simulink model "test_kin_odwrotnej"  (Simulink 7.7)
settings: Solver=FixedStepDiscrete  StartTime=0.0  StopTime=0  FixedStep=1  RelTol=1e-3
values from neighbouring files (symbols this model uses):
  Rmax = 947    [kin_odwr.mat]    (also in test_kin_odwr_ost.m = 945)
  Rmin = 461    [kin_odwr.mat]    (also in test_kin_odwr_ost.m = 463)
  wsp_x = 1010    [kin_odwr.mat]    (also in test_kin_odwr_ost.m = (j-100)*10)
  wsp_y = 2610    [kin_odwr.mat]    (also in test_kin_odwr_ost.m = (i-100)*10)
  wsp_z = 930    [kin_odwr.mat]    (also in test_kin_odwr.m; test_kin_odwr_ost.m)
  y_akt = 0    [kin_odwr.mat]    (also in test_kin_odwr_ost.m)
undefined symbols (not defined in the file or in its folder): sgn
libraries: simulink x27, simulink_extras x4
settings Model: Creator=Maciek  LastModifiedBy=Maciek

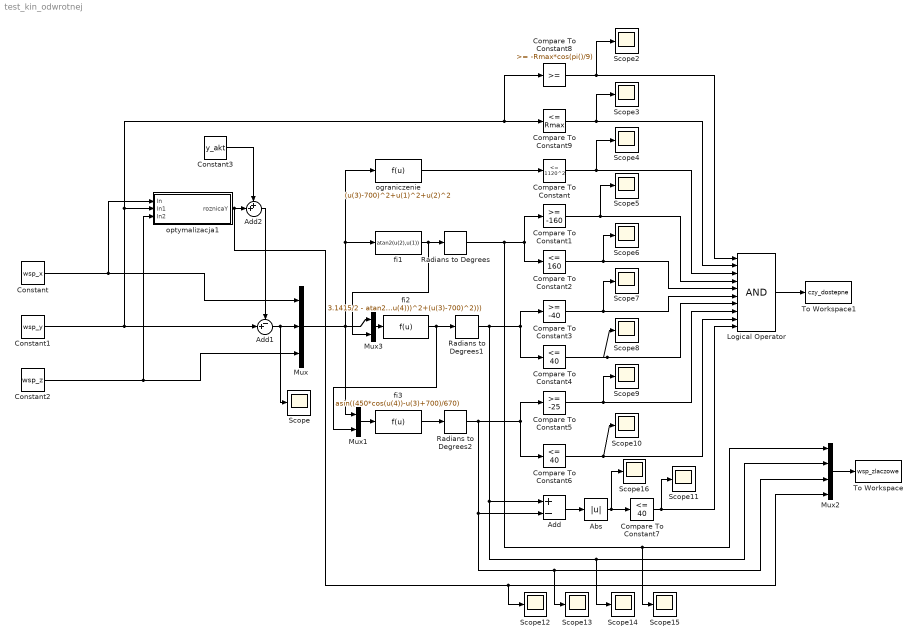
== system test_kin_odwrotnej ==
  Abs : Abs
  Add : Sum  Inputs=+-
  Add1 : Sum  Inputs=-+|
  Add2 : Sum  Inputs=++|
  Compare To Constant : simulink/Logic and Bit Operations/Compare To Constant  SystemSampleTime=-1  relop=<=  const=1120^2  LogicOutDataTypeMode=boolean  ZeroCross=off
  Compare To Constant1 : simulink/Logic and Bit Operations/Compare To Constant  SystemSampleTime=-1  relop=>=  const=-160  LogicOutDataTypeMode=boolean  ZeroCross=off
  Compare To Constant2 : simulink/Logic and Bit Operations/Compare To Constant  SystemSampleTime=-1  relop=<=  const=160  LogicOutDataTypeMode=boolean  ZeroCross=off
  Compare To Constant3 : simulink/Logic and Bit Operations/Compare To Constant  SystemSampleTime=-1  relop=>=  const=-40  LogicOutDataTypeMode=boolean  ZeroCross=off
  Compare To Constant4 : simulink/Logic and Bit Operations/Compare To Constant  SystemSampleTime=-1  relop=<=  const=40  LogicOutDataTypeMode=boolean  ZeroCross=off
  Compare To Constant5 : simulink/Logic and Bit Operations/Compare To Constant  SystemSampleTime=-1  relop=>=  const=-25  LogicOutDataTypeMode=boolean  ZeroCross=off
  Compare To Constant6 : simulink/Logic and Bit Operations/Compare To Constant  SystemSampleTime=-1  relop=<=  const=40  LogicOutDataTypeMode=boolean  ZeroCross=off
  Compare To Constant7 : simulink/Logic and Bit Operations/Compare To Constant  SystemSampleTime=-1  relop=<=  const=40  LogicOutDataTypeMode=boolean  ZeroCross=off
  Compare To Constant8 : simulink/Logic and Bit Operations/Compare To Constant  SystemSampleTime=-1  relop=>=  const=-Rmax*cos(pi()/9)  LogicOutDataTypeMode=boolean  ZeroCross=off
  Compare To Constant9 : simulink/Logic and Bit Operations/Compare To Constant  SystemSampleTime=-1  relop=<=  const=Rmax  LogicOutDataTypeMode=boolean  ZeroCross=off
  Constant : Constant  Value=wsp_x
  Constant1 : Constant  Value=wsp_y
  Constant2 : Constant  Value=wsp_z
  Constant3 : Constant  Value=y_akt  OutDataTypeStr=double
  Logical Operator : Logic  Inputs=10  AllPortsSameDT=off  OutDataTypeStr=boolean
  Mux : Mux  Inputs=3
  Mux1 : Mux  Inputs=2
  Mux2 : Mux
  Mux3 : Mux  Inputs=2
  Radians to Degrees : simulink_extras/Transformations/Radians to Degrees  SystemSampleTime=-1
  Radians to Degrees1 : simulink_extras/Transformations/Radians to Degrees  SystemSampleTime=-1
  Radians to Degrees2 : simulink_extras/Transformations/Radians to Degrees  SystemSampleTime=-1
  Scope{,2..16} (16 alike) : Scope
      Scope settings: SaveName=ScopeData18
      Scope10 settings: SaveName=ScopeData35
      Scope11 settings: SaveName=ScopeData36
      Scope12 settings: SaveName=ScopeData37
      Scope13 settings: SaveName=ScopeData38
      Scope14 settings: SaveName=ScopeData39
      Scope15 settings: SaveName=ScopeData40
      Scope16 settings: SaveName=ScopeData47
      Scope2 settings: SaveName=ScopeData27
      Scope3 settings: SaveName=ScopeData28
      Scope4 settings: SaveName=ScopeData29
      Scope5 settings: SaveName=ScopeData30
      Scope6 settings: SaveName=ScopeData31
      Scope7 settings: SaveName=ScopeData32
      Scope8 settings: SaveName=ScopeData33
      Scope9 settings: SaveName=ScopeData34
  To Workspace : ToWorkspace  VariableName=wsp_zlaczowe  SampleTime=-1  SaveFormat=Array
  To Workspace1 : ToWorkspace  VariableName=czy_dostepne  SampleTime=-1  SaveFormat=Array
  fi1 : Fcn  Expr=atan2(u(2),u(1))
  fi2 : Fcn  Expr=3.1415/2 - atan2((u(3)-700),sqrt((u(1)-cos(u(4))*250)^2+(u(2)-250*sin(u(4)))^2)) - acos((450^2+(u(1)-250*cos(u(4)))^2+(u(2)-250*sin(u(4)))^2+(u(3)-700)^2-670^2)/(2*450*sqrt((u(1)-250*cos(u(4)))^2+(u(2)-250*sin(u(4)))^2+(u(3)-700)^2)))
  fi3 : Fcn  Expr=asin((450*cos(u(4))-u(3)+700)/670)
  ograniczenie : Fcn  Expr=(u(3)-700)^2+u(1)^2+u(2)^2
  optymalizacja1 : Subsystem
  wires:
  fi1/1 -> Radians to Degrees/1, Mux3/2
  ograniczenie/1 -> Compare To Constant/1
  Radians to Degrees/1 -> Compare To Constant1/1, Compare To Constant2/1, Mux2/1, Scope15/1
  Add/1 -> Abs/1
  Abs/1 -> Compare To Constant7/1, Scope16/1
  Radians to Degrees1/1 -> Compare To Constant3/1, Compare To Constant4/1, Add/1, Mux2/2, Scope14/1
  fi3/1 -> Radians to Degrees2/1
  fi2/1 -> Radians to Degrees1/1, Mux1/2
  Radians to Degrees2/1 -> Compare To Constant5/1, Compare To Constant6/1, Add/2, Scope13/1, Mux2/3
  Compare To Constant7/1 -> Logical Operator/10, Scope11/1
  Compare To Constant/1 -> Logical Operator/3, Scope4/1
  Compare To Constant1/1 -> Logical Operator/4, Scope5/1
  Compare To Constant2/1 -> Logical Operator/5, Scope6/1
  Compare To Constant3/1 -> Logical Operator/6, Scope7/1
  Compare To Constant4/1 -> Logical Operator/7, Scope8/1
  Compare To Constant5/1 -> Logical Operator/8, Scope9/1
  Compare To Constant6/1 -> Logical Operator/9, Scope10/1
  Mux1/1 -> fi3/1
  Mux/1 -> ograniczenie/1, fi1/1, Mux1/1, Mux3/1
  Constant2/1 -> Mux/3, optymalizacja1/3(In2)
  Constant1/1 -> optymalizacja1/2(In1), Compare To Constant9/1, Compare To Constant8/1, Add1/2
  Compare To Constant9/1 -> Logical Operator/2, Scope3/1
  Compare To Constant8/1 -> Logical Operator/1, Scope2/1
  Mux2/1 -> To Workspace/1
  Constant/1 -> optymalizacja1/1(In), Mux/1
  Add1/1 -> Mux/2, Scope/1
  Logical Operator/1 -> To Workspace1/1
  optymalizacja1/1(roznicaY) -> Add2/2, Mux2/4, Scope12/1
  Add2/1 -> Add1/1
  Constant3/1 -> Add2/1
  Mux3/1 -> fi2/1

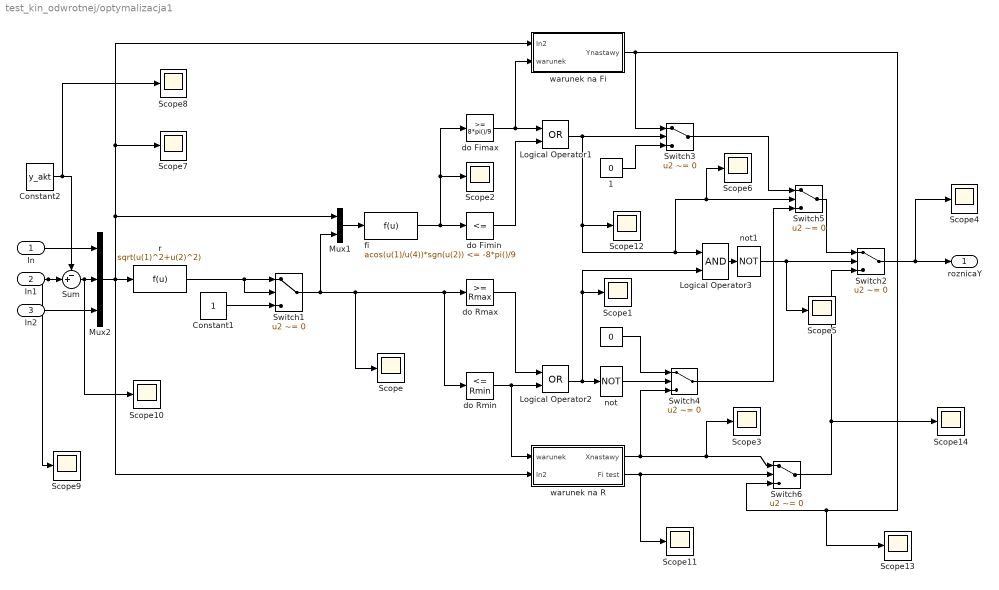
== system test_kin_odwrotnej/optymalizacja1 ==
  In : Inport
  In1 : Inport  Port=2
  In2 : Inport  Port=3
  " " : Constant  Value=0  OutDataTypeStr=double
  " 1" : Constant  Value=0  OutDataTypeStr=double
  Constant1 : Constant  OutDataTypeStr=double
  Constant2 : Constant  Value=y_akt  OutDataTypeStr=double
  Logical Operator1 : Logic  Operator=OR  AllPortsSameDT=off  OutDataTypeStr=boolean
  Logical Operator2 : Logic  Operator=OR  AllPortsSameDT=off  OutDataTypeStr=boolean
  Logical Operator3 : Logic  AllPortsSameDT=off  OutDataTypeStr=boolean
  Mux1 : Mux  Inputs=2
  Mux2 : Mux  Inputs=3
  Scope{,1..14} (15 alike) : Scope
      Scope10 settings: SaveName=ScopeData46
      Scope11 settings: SaveName=ScopeData50
      Scope12 settings: SaveName=ScopeData51
      Scope13 settings: SaveName=ScopeData53
      Scope14 settings: SaveName=ScopeData54
      Scope2 settings: SaveName=ScopeData2
      Scope3 settings: SaveName=ScopeData3
      Scope4 settings: SaveName=ScopeData16
      Scope5 settings: SaveName=ScopeData17
      Scope6 settings: SaveName=ScopeData41
      Scope7 settings: SaveName=ScopeData43
      Scope8 settings: SaveName=ScopeData44
      Scope9 settings: SaveName=ScopeData45
  Sum : Sum  Inputs=-+|
  Switch1 : Switch  Criteria=u2 ~= 0  OutDataTypeStr=double
  Switch{2..6} (5 alike) : Switch  Criteria=u2 ~= 0
  do Fimax : simulink/Logic and Bit Operations/Compare To Constant  SystemSampleTime=-1  relop=>=  const=8*pi()/9  LogicOutDataTypeMode=uint8  ZeroCross=off
  do Fimin : simulink/Logic and Bit Operations/Compare To Constant  SystemSampleTime=-1  relop=<=  const=-8*pi()/9  LogicOutDataTypeMode=uint8  ZeroCross=off
  do Rmax : simulink/Logic and Bit Operations/Compare To Constant  SystemSampleTime=-1  relop=>=  const=Rmax  LogicOutDataTypeMode=uint8  ZeroCross=off
  do Rmin : simulink/Logic and Bit Operations/Compare To Constant  SystemSampleTime=-1  relop=<=  const=Rmin  LogicOutDataTypeMode=uint8  ZeroCross=off
  fi : Fcn  Expr=acos(u(1)/u(4))*sgn(u(2))
  not : Logic  Operator=NOT  AllPortsSameDT=off  OutDataTypeStr=boolean
  not1 : Logic  Operator=NOT  AllPortsSameDT=off  OutDataTypeStr=boolean
  r : Fcn  Expr=sqrt(u(1)^2+u(2)^2)
  warunek na Fi : Subsystem  TreatAsAtomicUnit=on
  warunek na R : Subsystem  TreatAsAtomicUnit=on
  roznicaY : Outport
  wires:
  Switch6/1 -> Switch2/3, Scope14/1
  warunek na R/2(Fi test) -> Switch6/2, Scope11/1
  not1/1 -> Switch2/2, Scope5/1
  Switch3/1 -> Switch5/1
  Switch4/1 -> Switch5/3
  Switch5/1 -> Switch2/1
  Logical Operator3/1 -> not1/1
  " 1"/1 -> Switch3/3
  " "/1 -> Switch4/1
  not/1 -> Switch4/2
  warunek na R/1(Xnastawy) -> Switch4/3, Switch6/1, Scope3/1
  warunek na Fi/1(Ynastawy) -> Switch3/1, Switch6/3, Scope13/1
  Logical Operator1/1 -> Switch3/2, Logical Operator3/1, Switch5/2, Scope6/1, Scope12/1
  Logical Operator2/1 -> not/1, Logical Operator3/2, Scope1/1
  do Rmin/1 -> Logical Operator2/2, warunek na R/1(warunek)
  do Rmax/1 -> Logical Operator2/1
  do Fimin/1 -> Logical Operator1/2
  do Fimax/1 -> warunek na Fi/2(warunek), Logical Operator1/1
  fi/1 -> do Fimin/1, do Fimax/1, Scope2/1
  Constant1/1 -> Switch1/3
  Mux1/1 -> fi/1
  Switch1/1 -> Mux1/2, do Rmax/1, do Rmin/1, Scope/1
  r/1 -> Switch1/2, Switch1/1
  Mux2/1 -> r/1, Mux1/1, warunek na Fi/1(In2), Scope7/1, warunek na R/2(In2)
  In/1 -> Mux2/1
  In2/1 -> Mux2/3
  Switch2/1 -> roznicaY/1, Scope4/1
  Sum/1 -> Mux2/2, Scope10/1
  In1/1 -> Sum/2, Scope9/1
  Constant2/1 -> Sum/1, Scope8/1

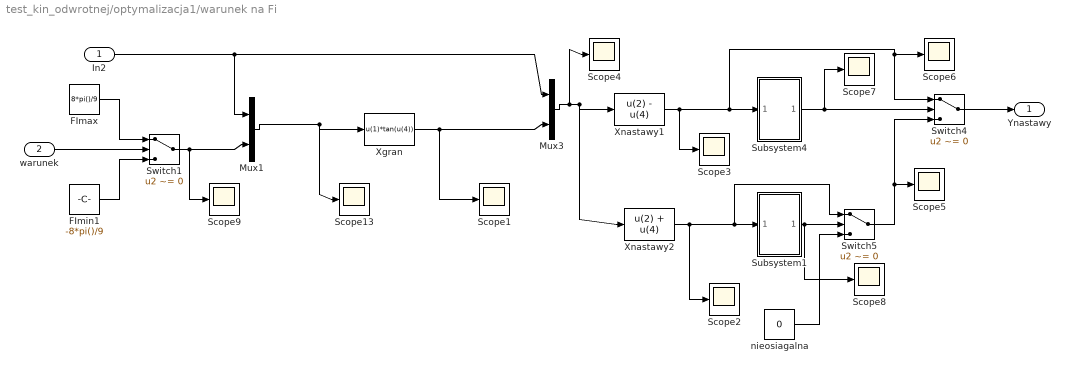
== system test_kin_odwrotnej/optymalizacja1/warunek na Fi ==
  In2 : Inport
  warunek : Inport  Port=2
  FImax : Constant  Value=8*pi()/9  OutDataTypeStr=double
      settings: SamplingMode=Frame based
  FImin1 : Constant  Value=-8*pi()/9  OutDataTypeStr=double
      settings: SamplingMode=Frame based
  Mux1 : Mux  Inputs=2
  Mux3 : Mux  Inputs=2
  Scope{1..9,13} (10 alike) : Scope
      Scope1 settings: SaveName=ScopeData56
      Scope13 settings: SaveName=ScopeData55
      Scope2 settings: SaveName=ScopeData57
      Scope3 settings: SaveName=ScopeData58
      Scope4 settings: SaveName=ScopeData59
      Scope5 settings: SaveName=ScopeData60
      Scope6 settings: SaveName=ScopeData61
      Scope7 settings: SaveName=ScopeData62
      Scope8 settings: SaveName=ScopeData63
      Scope9 settings: SaveName=ScopeData64
  Subsystem1 : Subsystem
  Subsystem4 : Subsystem
  Switch1 : Switch  Criteria=u2 ~= 0  OutDataTypeStr=double
  Switch4 : Switch  Criteria=u2 ~= 0
  Switch5 : Switch  Criteria=u2 ~= 0
  Xgran : Fcn  Expr=u(1)*tan(u(4))
  Xnastawy1 : Fcn  Expr=u(2) - u(4)
  Xnastawy2 : Fcn  Expr=u(2) + u(4)
  nieosiagalna : Constant  Value=0  OutDataTypeStr=double
  Ynastawy : Outport
  wires:
  Xgran/1 -> Scope1/1, Mux3/2
  FImax/1 -> Switch1/1
  Mux1/1 -> Xgran/1, Scope13/1
  Mux3/1 -> Xnastawy1/1, Xnastawy2/1, Scope4/1
  Subsystem4/1(Out1) -> Switch4/2, Scope7/1
  Switch5/1 -> Switch4/3, Scope5/1
  Subsystem1/1(Out1) -> Switch5/2, Scope8/1
  nieosiagalna/1 -> Switch5/3
  Switch4/1 -> Ynastawy/1
  Xnastawy1/1 -> Subsystem4/1(In1), Switch4/1, Scope6/1, Scope3/1
  Xnastawy2/1 -> Switch5/1, Subsystem1/1(In1), Scope2/1
  In2/1 -> Mux1/1, Mux3/1
  Switch1/1 -> Scope9/1, Mux1/2
  warunek/1 -> Switch1/2
  FImin1/1 -> Switch1/3

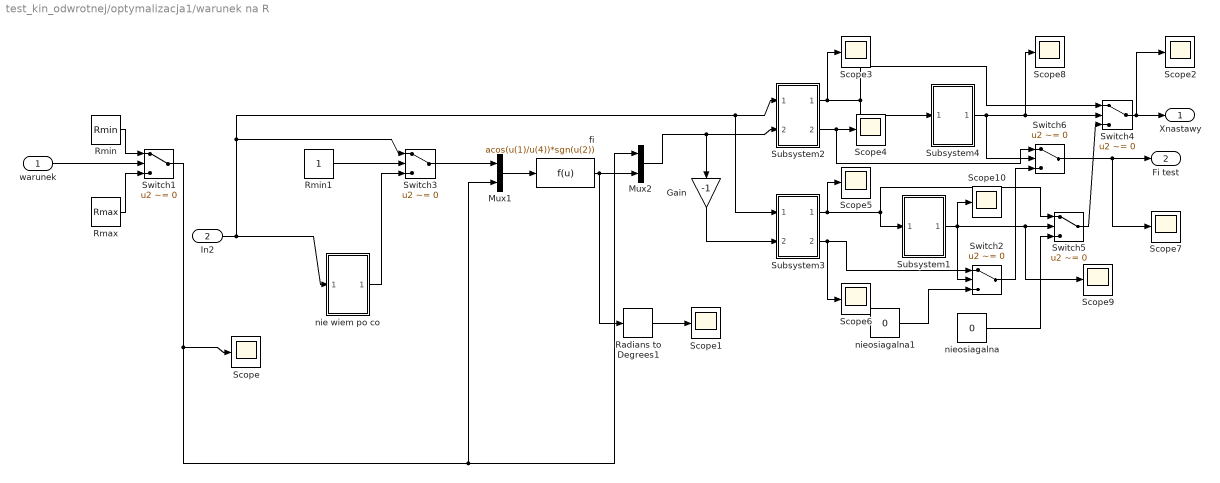
== system test_kin_odwrotnej/optymalizacja1/warunek na R ==
  warunek : Inport
  In2 : Inport  Port=2
  Gain : Gain  Gain=-1
  Mux1 : Mux  Inputs=2
  Mux2 : Mux  Inputs=2
  Radians to Degrees1 : simulink_extras/Transformations/Radians to Degrees  SystemSampleTime=-1
  Rmax : Constant  Value=Rmax  OutDataTypeStr=double
  Rmin : Constant  Value=Rmin  OutDataTypeStr=double
  Rmin1 : Constant  OutDataTypeStr=boolean
  Scope{,1..10} (11 alike) : Scope
      Scope settings: SaveName=ScopeData4
      Scope1 settings: SaveName=ScopeData5
      Scope10 settings: SaveName=ScopeData49
      Scope2 settings: SaveName=ScopeData14
      Scope3 settings: SaveName=ScopeData7
      Scope4 settings: SaveName=ScopeData8
      Scope5 settings: TimeRange=1  SaveName=ScopeData9
      Scope6 settings: SaveName=ScopeData10
      Scope7 settings: SaveName=ScopeData15
      Scope8 settings: SaveName=ScopeData21
      Scope9 settings: SaveName=ScopeData48
  Subsystem1 : Subsystem
  Subsystem2 : Subsystem
  Subsystem3 : Subsystem
  Subsystem4 : Subsystem
  Switch{1..6} (6 alike) : Switch  Criteria=u2 ~= 0
  fi : Fcn  Expr=acos(u(1)/u(4))*sgn(u(2))
  nie wiem po co : Subsystem
  nieosiagalna : Constant  Value=0  OutDataTypeStr=double
  nieosiagalna1 : Constant  Value=0  OutDataTypeStr=double
  Xnastawy : Outport
  Fi test : Outport  Port=2
  wires:
  fi/1 -> Mux2/2, Radians to Degrees1/1
  Mux1/1 -> fi/1
  In2/1 -> nie wiem po co/1(In1), Subsystem3/1(In2), Subsystem2/1(In2), Switch3/1
  Switch1/1 -> Mux1/2, Mux2/1, Scope/1
  warunek/1 -> Switch1/2
  Subsystem4/1(Out1) -> Switch6/2, Switch4/2, Scope8/1
  Switch5/1 -> Switch4/3
  Subsystem1/1(Out1) -> Switch2/2, Switch5/2, Scope9/1, Scope10/1
  nieosiagalna/1 -> Switch5/3
  Mux2/1 -> Subsystem2/2(In3), Gain/1
  Switch6/1 -> Fi test/1, Scope7/1
  Switch4/1 -> Xnastawy/1, Scope2/1
  Gain/1 -> Subsystem3/2(In3)
  Subsystem3/1(Out1) -> Switch5/1, Subsystem1/1(In1), Scope5/1
  Subsystem3/2(Out2) -> Switch2/1, Scope6/1
  Subsystem2/1(Out1) -> Subsystem4/1(In1), Switch4/1, Scope3/1
  Subsystem2/2(Out2) -> Switch6/1, Scope4/1
  Switch2/1 -> Switch6/3
  nieosiagalna1/1 -> Switch2/3
  nie wiem po co/1(Out1) -> Switch3/3
  Switch3/1 -> Mux1/1
  Rmin1/1 -> Switch3/2
  Radians to Degrees1/1 -> Scope1/1
  Rmin/1 -> Switch1/1
  Rmax/1 -> Switch1/3

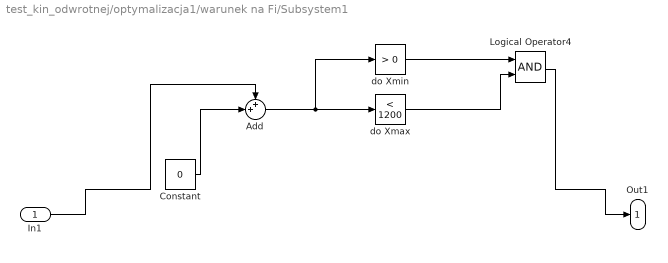
== system test_kin_odwrotnej/optymalizacja1/warunek na Fi/Subsystem1 ==
  In1 : Inport
  Add : Sum  Inputs=++|
  Constant : Constant  Value=0
  Logical Operator4 : Logic  AllPortsSameDT=off  OutDataTypeStr=boolean
  do Xmax : simulink/Logic and Bit Operations/Compare To Constant  SystemSampleTime=-1  relop=<  const=1200  LogicOutDataTypeMode=uint8  ZeroCross=off
  do Xmin : simulink/Logic and Bit Operations/Compare To Constant  SystemSampleTime=-1  relop=>  const=0  LogicOutDataTypeMode=uint8  ZeroCross=off
  Out1 : Outport
  wires:
  In1/1 -> Add/1
  Logical Operator4/1 -> Out1/1
  Add/1 -> do Xmax/1, do Xmin/1
  Constant/1 -> Add/2
  do Xmax/1 -> Logical Operator4/2
  do Xmin/1 -> Logical Operator4/1

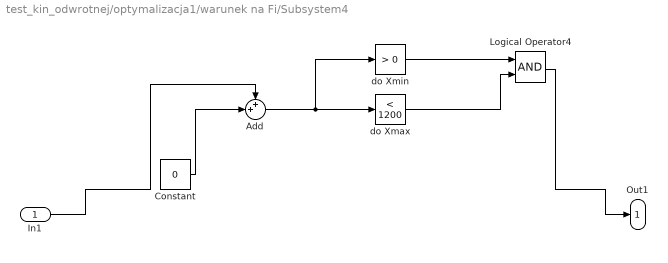
== system test_kin_odwrotnej/optymalizacja1/warunek na Fi/Subsystem4 ==
  In1 : Inport
  Add : Sum  Inputs=++|
  Constant : Constant  Value=0
  Logical Operator4 : Logic  AllPortsSameDT=off  OutDataTypeStr=boolean
  do Xmax : simulink/Logic and Bit Operations/Compare To Constant  SystemSampleTime=-1  relop=<  const=1200  LogicOutDataTypeMode=uint8  ZeroCross=off
  do Xmin : simulink/Logic and Bit Operations/Compare To Constant  SystemSampleTime=-1  relop=>  const=0  LogicOutDataTypeMode=uint8  ZeroCross=off
  Out1 : Outport
  wires:
  do Xmin/1 -> Logical Operator4/1
  do Xmax/1 -> Logical Operator4/2
  Constant/1 -> Add/2
  Add/1 -> do Xmin/1, do Xmax/1
  Logical Operator4/1 -> Out1/1
  In1/1 -> Add/1

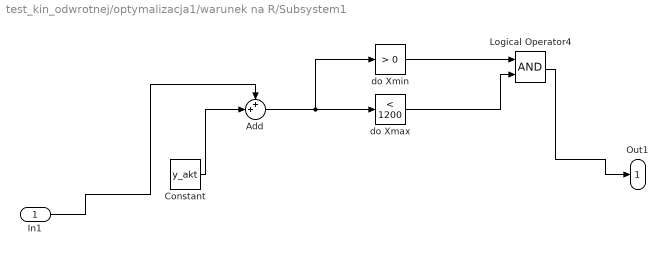
== system test_kin_odwrotnej/optymalizacja1/warunek na R/Subsystem1 ==
  In1 : Inport
  Add : Sum  Inputs=++|
  Constant : Constant  Value=y_akt
  Logical Operator4 : Logic  AllPortsSameDT=off  OutDataTypeStr=boolean
  do Xmax : simulink/Logic and Bit Operations/Compare To Constant  SystemSampleTime=-1  relop=<  const=1200  LogicOutDataTypeMode=uint8  ZeroCross=off
  do Xmin : simulink/Logic and Bit Operations/Compare To Constant  SystemSampleTime=-1  relop=>  const=0  LogicOutDataTypeMode=uint8  ZeroCross=off
  Out1 : Outport
  wires:
  In1/1 -> Add/1
  Logical Operator4/1 -> Out1/1
  Add/1 -> do Xmax/1, do Xmin/1
  Constant/1 -> Add/2
  do Xmax/1 -> Logical Operator4/2
  do Xmin/1 -> Logical Operator4/1

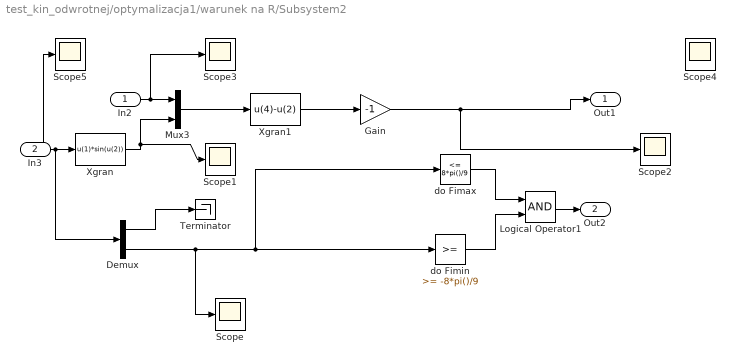
== system test_kin_odwrotnej/optymalizacja1/warunek na R/Subsystem2 ==
  In2 : Inport
  In3 : Inport  Port=2
  Demux : Demux  Outputs=2
  Gain : Gain  Gain=-1
  Logical Operator1 : Logic  AllPortsSameDT=off  OutDataTypeStr=boolean
  Mux3 : Mux  Inputs=2
  Scope{,1..5} (6 alike) : Scope
      Scope settings: SaveName=ScopeData6
      Scope1 settings: SaveName=ScopeData11
      Scope2 settings: SaveName=ScopeData12
      Scope3 settings: SaveName=ScopeData13
      Scope4 settings: SaveName=ScopeData20
      Scope5 settings: SaveName=ScopeData42
  Terminator : Terminator
  Xgran : Fcn  Expr=u(1)*sin(u(2))
  Xgran1 : Fcn  Expr=u(4)-u(2)
  do Fimax : simulink/Logic and Bit Operations/Compare To Constant  SystemSampleTime=-1  relop=<=  const=8*pi()/9  LogicOutDataTypeMode=uint8  ZeroCross=off
  do Fimin : simulink/Logic and Bit Operations/Compare To Constant  SystemSampleTime=-1  relop=>=  const=-8*pi()/9  LogicOutDataTypeMode=uint8  ZeroCross=off
  Out1 : Outport
  Out2 : Outport  Port=2
  wires:
  do Fimin/1 -> Logical Operator1/2
  do Fimax/1 -> Logical Operator1/1
  Xgran/1 -> Mux3/2, Scope1/1
  Mux3/1 -> Xgran1/1
  In2/1 -> Mux3/1, Scope3/1
  In3/1 -> Xgran/1, Demux/1, Scope5/1
  Logical Operator1/1 -> Out2/1
  Demux/2 -> do Fimin/1, do Fimax/1, Scope/1
  Demux/1 -> Terminator/1
  Xgran1/1 -> Gain/1
  Gain/1 -> Scope2/1, Out1/1

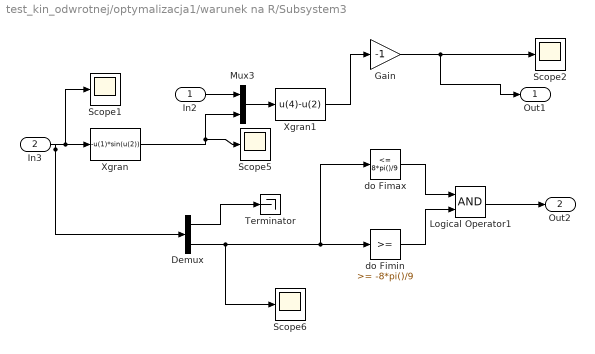
== system test_kin_odwrotnej/optymalizacja1/warunek na R/Subsystem3 ==
  In2 : Inport
  In3 : Inport  Port=2
  Demux : Demux  Outputs=2
  Gain : Gain  Gain=-1
  Logical Operator1 : Logic  AllPortsSameDT=off  OutDataTypeStr=boolean
  Mux3 : Mux  Inputs=2
  Scope{1..2,5..6} (4 alike) : Scope
      Scope1 settings: TimeRange=1  SaveName=ScopeData23
      Scope2 settings: TimeRange=1  SaveName=ScopeData24
      Scope5 settings: TimeRange=1  SaveName=ScopeData22
      Scope6 settings: TimeRange=1  SaveName=ScopeData52
  Terminator : Terminator
  Xgran : Fcn  Expr=-u(1)*sin(u(2))
  Xgran1 : Fcn  Expr=u(4)-u(2)
  do Fimax : simulink/Logic and Bit Operations/Compare To Constant  SystemSampleTime=-1  relop=<=  const=8*pi()/9  LogicOutDataTypeMode=uint8  ZeroCross=off
  do Fimin : simulink/Logic and Bit Operations/Compare To Constant  SystemSampleTime=-1  relop=>=  const=-8*pi()/9  LogicOutDataTypeMode=uint8  ZeroCross=off
  Out1 : Outport
  Out2 : Outport  Port=2
  wires:
  Logical Operator1/1 -> Out2/1
  In3/1 -> Xgran/1, Scope1/1, Demux/1
  In2/1 -> Mux3/1
  Mux3/1 -> Xgran1/1
  Xgran1/1 -> Gain/1
  Xgran/1 -> Mux3/2, Scope5/1
  do Fimax/1 -> Logical Operator1/1
  do Fimin/1 -> Logical Operator1/2
  Demux/2 -> do Fimin/1, do Fimax/1, Scope6/1
  Demux/1 -> Terminator/1
  Gain/1 -> Out1/1, Scope2/1

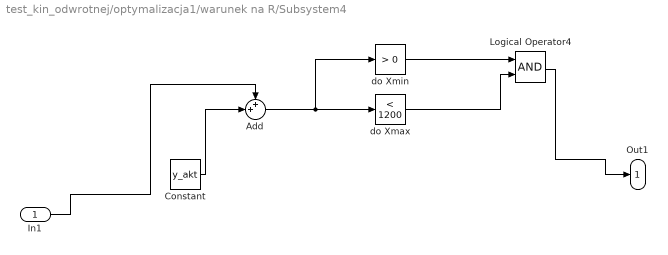
== system test_kin_odwrotnej/optymalizacja1/warunek na R/Subsystem4 ==
  In1 : Inport
  Add : Sum  Inputs=++|
  Constant : Constant  Value=y_akt
  Logical Operator4 : Logic  AllPortsSameDT=off  OutDataTypeStr=boolean
  do Xmax : simulink/Logic and Bit Operations/Compare To Constant  SystemSampleTime=-1  relop=<  const=1200  LogicOutDataTypeMode=uint8  ZeroCross=off
  do Xmin : simulink/Logic and Bit Operations/Compare To Constant  SystemSampleTime=-1  relop=>  const=0  LogicOutDataTypeMode=uint8  ZeroCross=off
  Out1 : Outport
  wires:
  do Xmin/1 -> Logical Operator4/1
  do Xmax/1 -> Logical Operator4/2
  Constant/1 -> Add/2
  Add/1 -> do Xmin/1, do Xmax/1
  Logical Operator4/1 -> Out1/1
  In1/1 -> Add/1

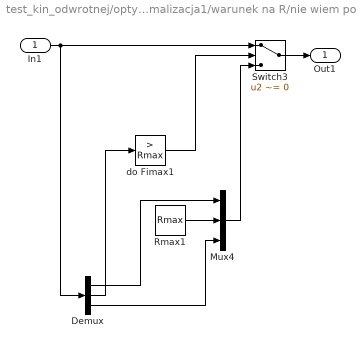
== system test_kin_odwrotnej/optymalizacja1/warunek na R/nie wiem po co ==
  In1 : Inport
  Demux : Demux  Outputs=3
  Mux4 : Mux  Inputs=3
  Rmax1 : Constant  Value=Rmax  OutDataTypeStr=double
  Switch3 : Switch  Criteria=u2 ~= 0
  do Fimax1 : simulink/Logic and Bit Operations/Compare To Constant  SystemSampleTime=-1  relop=>  const=Rmax  LogicOutDataTypeMode=boolean  ZeroCross=off
  Out1 : Outport
  wires:
  Demux/1 -> Mux4/1
  Demux/3 -> Mux4/3
  Demux/2 -> do Fimax1/1
  do Fimax1/1 -> Switch3/2
  Rmax1/1 -> Mux4/2
  Mux4/1 -> Switch3/3
  In1/1 -> Switch3/1, Demux/1
  Switch3/1 -> Out1/1
